simulink model "EKF1"  (R2024a)
settings: Solver=VariableStepAuto  StartTime=0.0  StopTime=10.0  RelTol=1e-3
settings Model: Creator=SHARI  LastModifiedBy=SHARI

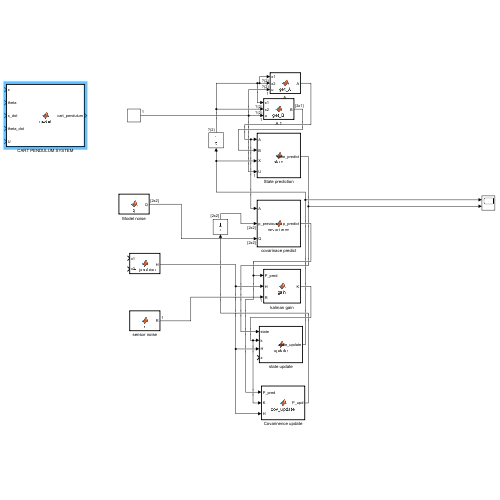
[thumbnail: Simulink's stored preview of the top-level diagram]
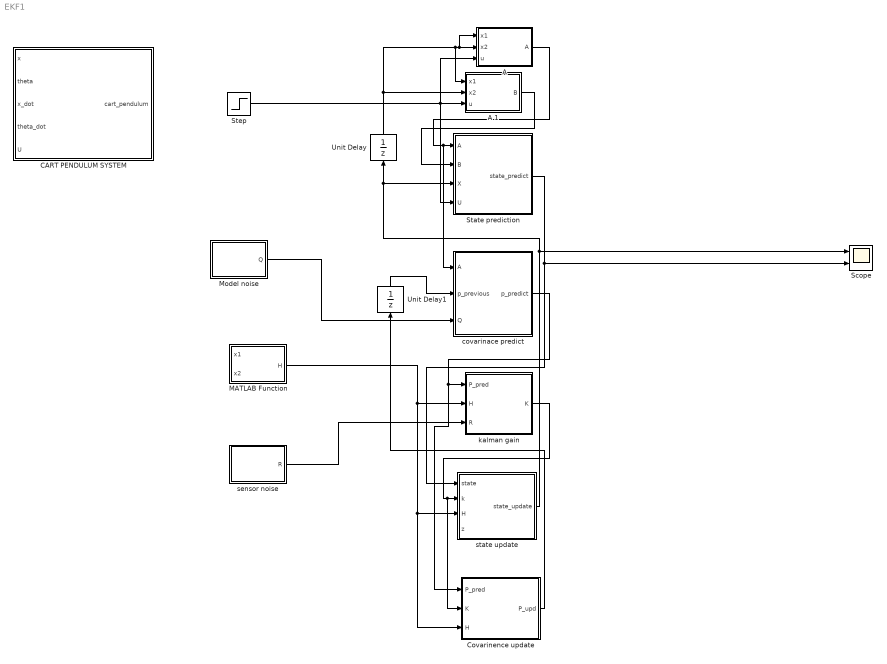
== system EKF1 ==
  "A " : MATLAB Function  TreatAsAtomicUnit=on
  A 1 : MATLAB Function  TreatAsAtomicUnit=on
  CART PENDULUM SYSTEM : MATLAB Function  TreatAsAtomicUnit=on
  Covarinence update : MATLAB Function  TreatAsAtomicUnit=on
  MATLAB Function : MATLAB Function  TreatAsAtomicUnit=on
  Model noise : MATLAB Function  TreatAsAtomicUnit=on
  Scope : Scope  NumInputPorts=2
  State prediction : MATLAB Function  TreatAsAtomicUnit=on
  Step : Step  SampleTime=0
  Unit Delay : UnitDelay  InitialCondition=[0;0]  SampleTime=-1  HasFrameUpgradeWarning=on
  Unit Delay1 : UnitDelay  InitialCondition=[1 0.01; 0.01 1]  SampleTime=-1  HasFrameUpgradeWarning=on
  covarinace predict : MATLAB Function  TreatAsAtomicUnit=on
  kalman gain : MATLAB Function  TreatAsAtomicUnit=on
  sensor noise : MATLAB Function  TreatAsAtomicUnit=on
  state update : MATLAB Function  TreatAsAtomicUnit=on
  wires:
  State prediction/1(state_predict) -> Scope/2, state update/1(state)
  state update/1(state_update) -> Scope/1, State prediction/3(X), Unit Delay/1
  Unit Delay/1 -> A 1/1(x1), "A "/2(x2), "A "/1(x1), A 1/2(x2)
  covarinace predict/1(p_predict) -> Covarinence update/1(P_pred), kalman gain/1(P_pred)
  Unit Delay1/1 -> covarinace predict/2(p_previous)
  Model noise/1(Q) -> covarinace predict/3(Q)
  MATLAB Function/1(H) -> state update/3(H), Covarinence update/3(H), kalman gain/2(H)
  kalman gain/1(K) -> Covarinence update/2(K), state update/2(k)
  Covarinence update/1(P_upd) -> Unit Delay1/1
  sensor noise/1(R) -> kalman gain/3(R)
  "A "/1(A) -> covarinace predict/1(A), State prediction/1(A)
  Step/1 -> State prediction/4(U), A 1/3(u), "A "/3(u)
  A 1/1(B) -> State prediction/2(B)

== matlab function EKF1/State prediction ==
  data: A input; B input; X input; U input; state_predict output
function state_predict=state(A, B, X, U)
    state_predict = A * X + B * U;
end

== matlab function EKF1/A  ==
  data: x1 input; x2 input; u input; A output
function A = get_A(x1, x2, u)
%#codegen
A = A_jacobian(x1, x2, u);
end

== matlab function EKF1/covarinace predict ==
  data: A input; p_predict output; p_previous input; Q input
function p_predict = covariance(A, p_previous, Q)
     P_pred = A * P_prev * A' + Q;
end

== matlab function EKF1/MATLAB Function ==
  data: H output; x1 input; x2 input
function H = H_jacobian(x1, x2)
    syms x1 x2 real
    x = [x1; x2];

    % Define your measurement model h(x)
    h = [x1];  % change this based on what your sensor measures

    % Jacobian of h(x) w.r.t. x
    H = jacobian(h, x);
end

== matlab function EKF1/kalman gain ==
  data: P_pred input; K output; H input; R input
function K = gain(P_pred, H, R)
    K = P_pred * H' / (H * P_pred * H' + R);
end

== matlab function EKF1/state update ==
  data: state input; state_update output; k input; H input; z input
function state_update = update(state, k, H, z)
    state_update = state + k * (z - H * state);
end

== matlab function EKF1/Covarinence update ==
  data: P_pred input; P_upd output; K input; H input
function P_upd = cov_update(P_pred, K, H)
    I = eye(size(P_pred));
    P_upd = (I - K * H) * P_pred;
end

== matlab function EKF1/Model noise ==
  data: Q output
function Q  = q
Q = [0.001 0; 0 0.001];
end

== matlab function EKF1/sensor noise ==
  data: R output
function R = r()
R = 0.5;
end

== matlab function EKF1/CART PENDULUM SYSTEM ==
  data: x input; cart_pendulum output; theta input; x_dot input; theta_dot input; U input
function cart_pendulum = model(x, theta, x_dot, theta_dot, U)
 % Parameters (you can also make these inputs if needed)
    mc = 1.0;    % cart mass
    mp = 0.1;    % pendulum mass
    L = 0.5;     % pendulum length to CoM
    g = 9.81;    % gravity
    I = 0.006;

    D = [mp + mc -mp*cos(theta) * L; -mp*cos(theta) * L (I + mp * L^2)];
    C = [-mp * sin(theta) * theta_dot; 0];
    G = [0 ; -mp * L *sin(theta)]
    U = [1; 0];

    q     = [x; theta];
    q_dot = [x_dot; theta_dot];

     q_ddot = D \ (H*u - Cqdot - G);

       cart_pendulum = [x_dot;
          q_ddot(1);
          theta_dot;
          q_ddot(2)];
end

== matlab function EKF1/A 1 ==
  data: x1 input; x2 input; u input; B output
function B = get_B(x1, x2, u)
%#codegen
B = B_jacobian(x1, x2, u);
end
